simulink model "motor_model_ss"  (R2015a)
settings: Solver=ode45  StartTime=0.0  StopTime=10.0  RelTol=1e-3
undefined symbols (not defined in the file or in its folder): C1, C2, Kf, R, Ra
settings Model: Creator=Paul  LastModifiedBy=miguel

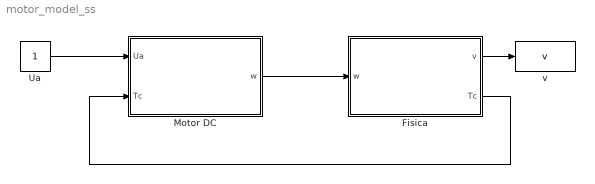
== system motor_model_ss ==
  Fisica : Subsystem
  Motor DC : Subsystem
  Ua : Constant
  v : ToWorkspace  VariableName=v  SampleTime=-1
  wires:
  Ua/1 -> Motor DC/1("Ua ")
  Motor DC/1(w) -> Fisica/1(w)
  Fisica/2(Tc) -> Motor DC/2(Tc)
  Fisica/1(v) -> v/1

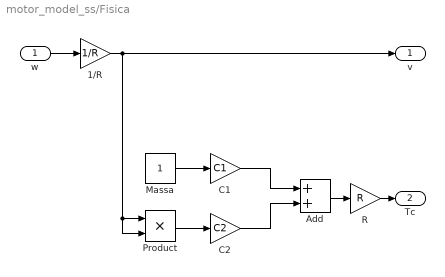
== system motor_model_ss/Fisica ==
  w : Inport
  1/R : Gain  Gain=1/R
  Add : Sum
  C1 : Gain  Gain=C1
  C2 : Gain  Gain=C2
  Massa : Constant
  Product : Product
  R : Gain  Gain=R
  v : Outport
  Tc : Outport  Port=2
  wires:
  1/R/1 -> Product/1, Product/2, v/1
  w/1 -> 1/R/1
  R/1 -> Tc/1
  Add/1 -> R/1
  Product/1 -> C2/1
  C2/1 -> Add/2
  Massa/1 -> C1/1
  C1/1 -> Add/1

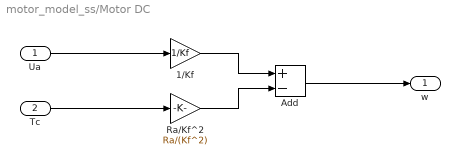
== system motor_model_ss/Motor DC ==
  "Ua " : Inport
  Tc : Inport  Port=2
  1/Kf : Gain  Gain=1/Kf
  Add : Sum  Inputs=+-
  Ra/Kf^2 : Gain  Gain=Ra/(Kf^2)
  w : Outport
  wires:
  "Ua "/1 -> 1/Kf/1
  Tc/1 -> Ra/Kf^2/1
  1/Kf/1 -> Add/1
  Ra/Kf^2/1 -> Add/2
  Add/1 -> w/1
